simulink model "ep_p_4_34"  (R2023b)
settings: Solver=VariableStepAuto  StartTime=0.0  StopTime=1000  RelTol=1e-3
libraries: simulink x1
settings Model: Creator=86186  LastModifiedBy=86186

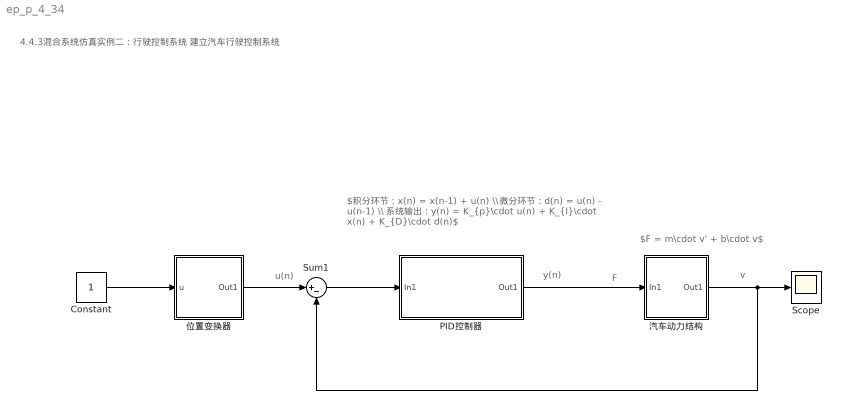
== system ep_p_4_34 ==
  note: $积分环节：x(n) = x(n-1) + u(n) \\ 微分环节：d(n) = u(n) - u(n-1) \\ 系统输出：y(n) = K_{p}\cdot u(n) + K_{I}\cdot x(n) + K_{D}\cdot d(n)$
  note: $F = m\cdot v' + b\cdot v$
  note: v
  note: F
  note: u(n)
  note: y(n)
  note: 4.4.3混合系统仿真实例二：行驶控制系统
      | 建立汽车行驶控制系统
  Constant : Constant
  PID控制器 : Subsystem
  Scope : Scope
  Sum1 : Sum  Inputs=|+-
  位置变换器 : Subsystem
  汽车动力结构 : Subsystem
  wires:
  Constant/1 -> 位置变换器/1(u)
  位置变换器/1(Out1) -> Sum1/1
  Sum1/1 -> PID控制器/1(In1)
  汽车动力结构/1(Out1) -> Scope/1, Sum1/2
  PID控制器/1(Out1) -> 汽车动力结构/1(In1)

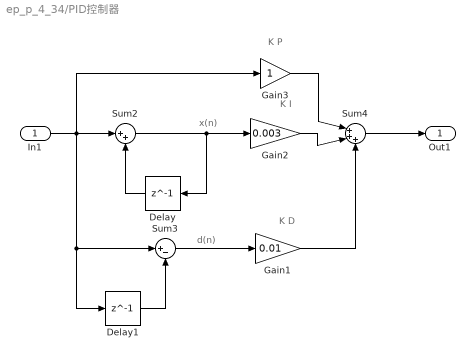
== system ep_p_4_34/PID控制器 ==
  note: x(n)
  note: K I
  note: K D
  note: d(n)
  note: K P
  In1 : Inport
  Delay : Delay  DelayLength=1  InitialCondition=0  SampleTime=0.02
  Delay1 : Delay  DelayLength=1  InitialCondition=0
  Gain1 : Gain  Gain=0.01
  Gain2 : Gain  Gain=0.003
  Gain3 : Gain
  Sum2 : Sum  Inputs=|++
  Sum3 : Sum  Inputs=|+-
  Sum4 : Sum  Inputs=|+++
  Out1 : Outport
  wires:
  Gain1/1 -> Sum4/3
  Delay1/1 -> Sum3/2
  Sum2/1 -> Delay/1, Gain2/1
  In1/1 -> Gain3/1, Delay1/1, Sum3/1, Sum2/1
  Gain3/1 -> Sum4/1
  Delay/1 -> Sum2/2
  Gain2/1 -> Sum4/2
  Sum3/1 -> Gain1/1
  Sum4/1 -> Out1/1

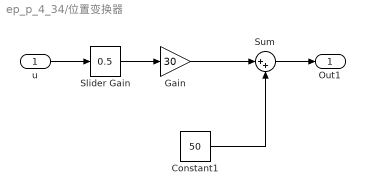
== system ep_p_4_34/位置变换器 ==
  u : Inport
  Constant1 : Constant  Value=50
  Gain : Gain  Gain=30
  Slider Gain : simulink/Math Operations/Slider Gain  gain=0.5  low=0  high=1
  Sum : Sum  Inputs=|++
  Out1 : Outport
  wires:
  Slider Gain/1 -> Gain/1
  u/1 -> Slider Gain/1
  Constant1/1 -> Sum/2
  Sum/1 -> Out1/1
  Gain/1 -> Sum/1

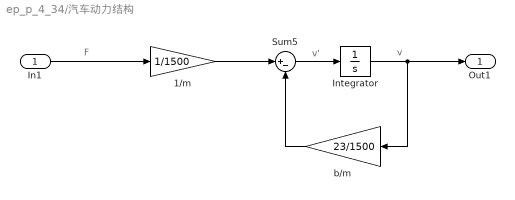
== system ep_p_4_34/汽车动力结构 ==
  note: F
  note: v
  note: v'
  In1 : Inport
  1/m : Gain  Gain=1/1500
  Integrator : Integrator
  Sum5 : Sum  Inputs=|+-
  b/m : Gain  Gain=23/1500
  Out1 : Outport
  wires:
  Sum5/1 -> Integrator/1
  1/m/1 -> Sum5/1
  Integrator/1 -> Out1/1, b/m/1
  In1/1 -> 1/m/1
  b/m/1 -> Sum5/2
